simulink model "KALMANC"  (R2019b)
settings: Solver=VariableStepAuto  StartTime=0.0  StopTime=10  RelTol=1e-3
values from neighbouring files (symbols this model uses):
  Ac = [(A-B*K)]    [State_Space.m]
  Bc = [B]    [State_Space.m]
  Cc = [C]    [State_Space.m]
  Dc = [D]    [State_Space.m]
  K = lqr(A,B,Q,R)    [LQG.m]    (also in State_Space.m; frequency_domain.m = 35; root_locus_method.m = 20; rscale.m = k)
  Nbar = rscale(sys_ss,K)    [State_Space.m]    (also in rscale.m = Nu + K*Nx)
undefined symbols (not defined in the file or in its folder): Ke
settings Model: Creator=Khojasteh Mirza  LastModifiedBy=Khojasteh Mirza

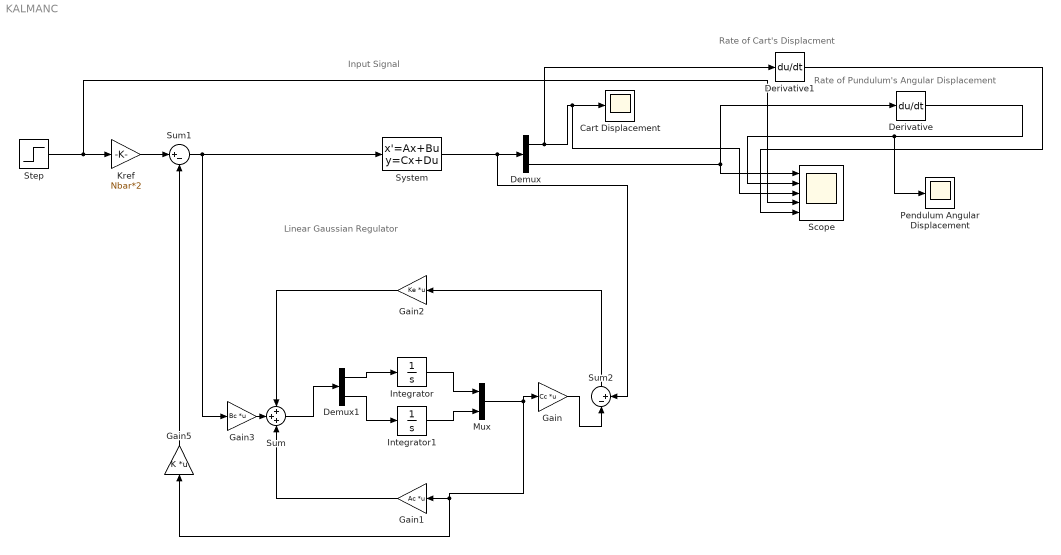
== system KALMANC ==
  note: Input Signal
  note: Rate of Pundulum's Angular Displacement
  note: Rate of Cart's Displacment
  note: Linear Gaussian Regulator
  "Cart Displacement " : Scope
  Demux : Demux  Outputs=2
  Demux1 : Demux  Outputs=2
  Derivative : Derivative
  Derivative1 : Derivative
  Gain : Gain  Gain=Cc  Multiplication=Matrix(K*u)
  Gain1 : Gain  Gain=Ac  Multiplication=Matrix(K*u)
  Gain2 : Gain  Gain=Ke  Multiplication=Matrix(K*u)
  Gain3 : Gain  Gain=Bc  Multiplication=Matrix(K*u)
  Gain5 : Gain  Gain=K  Multiplication=Matrix(K*u)
  Integrator : Integrator
  Integrator1 : Integrator
  Kref : Gain  Gain=Nbar*2
  Mux : Mux  Inputs=2
  Pendulum Angular Displacement : Scope
  Scope : Scope  NumInputPorts=5
  Step : Step  SampleTime=0
  Sum : Sum  Inputs=3
  Sum1 : Sum  Inputs=|+-
  Sum2 : Sum  Inputs=|-+
  System : StateSpace  A=Ac  B=Bc  C=Cc  D=Dc  InitialCondition=0
  wires:
  Integrator1/1 -> Mux/2
  System/1 -> Demux/1, Sum2/2
  Demux1/1 -> Integrator/1
  Gain1/1 -> Sum/3
  Sum/1 -> Demux1/1
  Gain3/1 -> Sum/2
  Kref/1 -> Sum1/1
  Sum1/1 -> Gain3/1, System/1
  Demux1/2 -> Integrator1/1
  Integrator/1 -> Mux/1
  Sum2/1 -> Gain2/1
  Mux/1 -> Gain/1, Gain5/1, Gain1/1
  Gain/1 -> Sum2/1
  Gain5/1 -> Sum1/2
  Gain2/1 -> Sum/1
  Demux/2 -> Derivative/1, Scope/1
  Demux/1 -> Derivative1/1, Scope/3, "Cart Displacement "/1
  Derivative/1 -> Pendulum Angular Displacement/1, Scope/2
  Derivative1/1 -> Scope/5
  Step/1 -> Scope/4, Kref/1
